simulink model "DCmotor_duo_PID_control_inter_position"  (R2023a)
settings: Solver=VariableStepAuto  StartTime=0.0  StopTime=inf  FixedStep=0.001  MaxStep=1e-3
values from neighbouring files (symbols this model uses):
  S = S_simple    [setupModelParameters.m]
undefined symbols (not defined in the file or in its folder): dval, ival, pval
libraries: slpidlib x1
settings Model: Creator=jamess  LastModifiedBy=leoyi
settings SolverCC: AlgebraicLoopSolver=TrustRegion
settings DataIOCC: ReturnWorkspaceOutputs=off
settings OptimizationCC: LifeSpan=inf
settings DebuggingCC: UnconnectedInputMsg=warning  UnconnectedOutputMsg=warning  UnconnectedLineMsg=warning  ArithmeticOperatorsInVariantConditions=warning
settings ModelReferenceCC: EnableRefExpFcnMdlSchedulingChecks=on
settings SFSimCC: SimUseLocalCustomCode=off  CustomCodeUndefinedFunction=UseInterfaceOnly
settings RTWCC: RTWUseLocalCustomCode=off
settings CodeAppCC: StateflowObjectComments=on

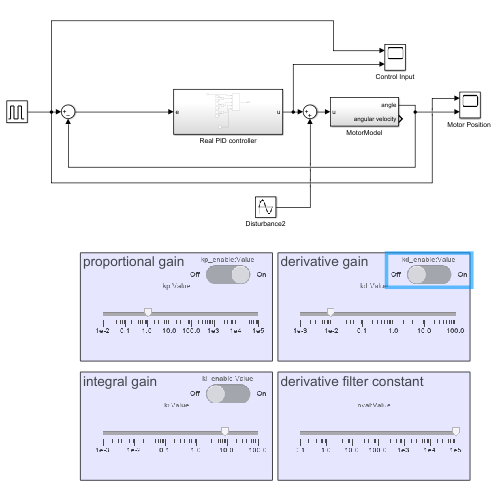
[thumbnail: Simulink's stored preview of the top-level diagram]
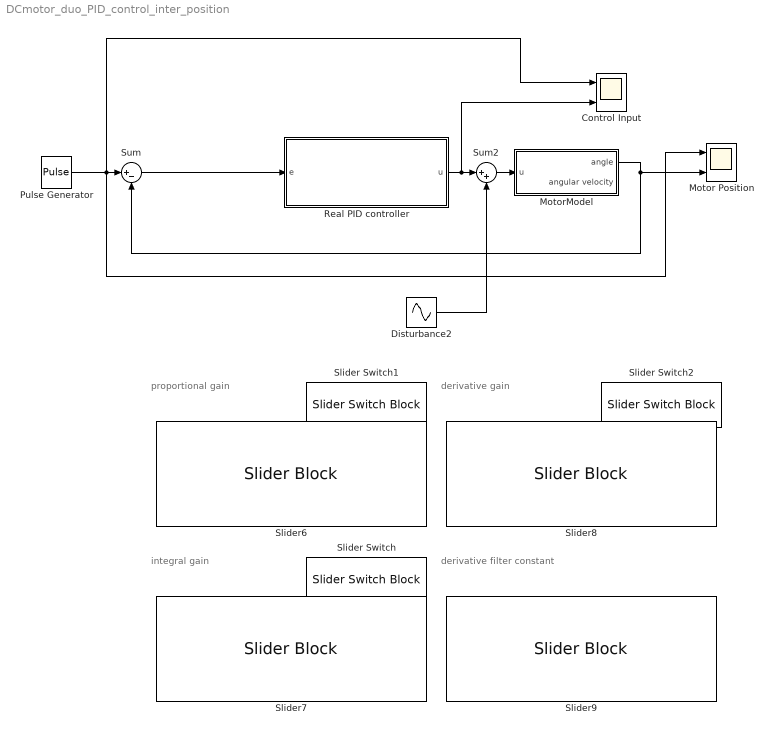
== system DCmotor_duo_PID_control_inter_position ==
  note: derivative gain
  note: proportional gain
  note: integral gain
  note: derivative filter constant
  Control Input : Scope  NumInputPorts=2
  Disturbance2 : Sin  Amplitude=0  Frequency=10*2*pi  SampleTime=0
  "Motor Position " : Scope  NumInputPorts=2
  MotorModel : Subsystem
  Pulse Generator : DiscretePulseGenerator  PulseType=Time based  Period=10  PulseWidth=50  PhaseDelay=0.1
  Real PID controller : Subsystem
  Slider Switch : SliderSwitchBlock
      settings: Values={{'Off', 'On'}, [0 1]}
  Slider Switch1 : SliderSwitchBlock
      settings: Values={{'Off', 'On'}, [0 1]}
  Slider Switch2 : SliderSwitchBlock
      settings: Values={{'Off', 'On'}, [0 1]}
  Slider6 : SliderBlock  ScaleMin=0.01  ScaleMax=100000  ScaleType=Log
  Slider7 : SliderBlock  ScaleMin=0.001  ScaleType=Log
  Slider8 : SliderBlock  ScaleMin=0.001  ScaleType=Log
  Slider9 : SliderBlock  ScaleMin=0.1  ScaleMax=1e5  ScaleType=Log
  Sum : Sum  Inputs=|+-
  Sum2 : Sum  Inputs=|++
  wires:
  MotorModel/1(angle) -> "Motor Position "/2, Sum/2
  Real PID controller/1(u) -> Control Input/2, Sum2/1
  Sum2/1 -> MotorModel/1(u)
  Pulse Generator/1 -> Control Input/1, "Motor Position "/1, Sum/1
  Disturbance2/1 -> Sum2/2
  Sum/1 -> Real PID controller/1(e)

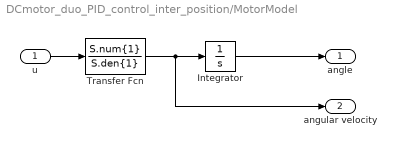
== system DCmotor_duo_PID_control_inter_position/MotorModel ==
  u : Inport
  Integrator : Integrator
  Transfer Fcn : TransferFcn  Numerator=S.num{1}  Denominator=S.den{1}
  angle : Outport
  angular velocity : Outport  Port=2
  wires:
  u/1 -> Transfer Fcn/1
  Transfer Fcn/1 -> angular velocity/1, Integrator/1
  Integrator/1 -> angle/1

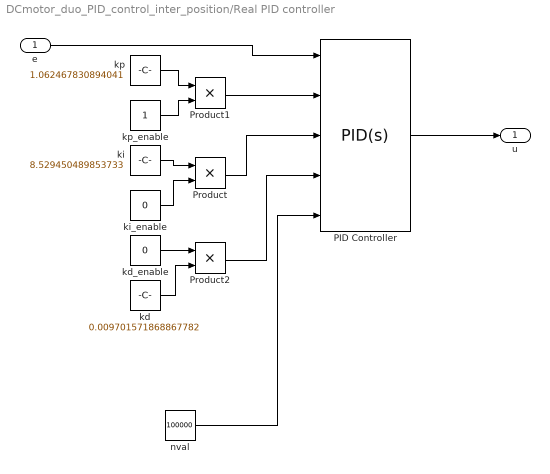
== system DCmotor_duo_PID_control_inter_position/Real PID controller ==
  e : Inport
  PID Controller : slpidlib/PID Controller  Controller=PID  Form=Parallel  TimeDomain=Continuous-time  UseExternalTs=off  SampleTime=-1  IntegratorMethod=Forward Euler  FilterMethod=Forward Euler  ControllerParametersSource=external  P=pval  I=ival  UseKiTs=off  D=dval  N=100  UseFilter=on  TunerSelectOption=Transfer Function Based (PID Tuner App)  InitialConditionSource=internal  InitialConditionForIntegrator=0  InitialConditionForFilter=0  DifferentiatorICPrevScaledInput=0  ExternalReset=none  TrackingMode=off  Kt=1  LimitOutput=off  SatLimitsSource=internal  UpperSaturationLimit=inf  LowerSaturationLimit=-inf  LinearizeAsGain=on  AntiWindupMode=none  Kb=1  LimitIntegrator=off  UpperIntegratorSaturationLimit=inf  LowerIntegratorSaturationLimit=-inf  POutMin=[]  POutMax=[]  IOutMin=[]  IOutMax=[]  DOutMin=[]  DOutMax=[]  NOutMin=[]  NOutMax=[]  SumOutMin=[]  SumOutMax=[]  SaturationOutMin=[]  SaturationOutMax=[]  PParamMin=[]  PParamMax=[]  IParamMin=[]  IParamMax=[]  DParamMin=[]  DParamMax=[]  NParamMin=[]  NParamMax=[]  KbParamMin=[]  KbParamMax=[]  KtParamMin=[]  KtParamMax=[]  KbOutMin=[]  KbOutMax=[]  KtOutMin=[]  KtOutMax=[]  IntegratorOutMin=[]  IntegratorOutMax=[]  FilterOutMin=[]  FilterOutMax=[]  SumI1OutMin=[]  SumI1OutMax=[]  SumI2OutMin=[]  SumI2OutMax=[]  SumI3OutMin=[]  SumI3OutMax=[]  SumI4OutMin=[]  SumI4OutMax=[]  SumDOutMin=[]  SumDOutMax=[]  DifferentiatorOutMin=[]  DifferentiatorOutMax=[]  FilterDiffOutCoefMin=[]  FilterDiffOutCoefMax=[]  ReciprocalOutMin=[]  ReciprocalOutMax=[]  SumDenOutMin=[]  SumDenOutMax=[]  SumNumOutMin=[]  SumNumOutMax=[]  DivideOutMin=[]  DivideOutMax=[]  UdiffTsProdOutMin=[]  UdiffTsProdOutMax=[]  NTsProdOutMin=[]  NTsProdOutMax=[]  UintegralTsProdOutMin=[]  UintegralTsProdOutMax=[]  UngainTsProdOutMin=[]  UngainTsProdOutMax=[]  ClampingZeroOutDataTypeStr=Inherit: Inherit via back propagation  ClampingZeroOutMin=[]  ClampingZeroOutMax=[]  FilterDenConstantOutDataTypeStr=Inherit: Inherit via back propagation  FilterDenConstantOutMin=[]  FilterDenConstantOutMax=[]  PCopyOutDataTypeStr=Inherit: Inherit via back propagation  PCopyOutMin=[]  PCopyOutMax=[]  NCopyOutDataTypeStr=Inherit: Inherit via back propagation  NCopyOutMin=[]  NCopyOutMax=[]  IntegratorContinuousStateAttributes=''  IntegratorStateMustResolveToSignalObject=off  IntegratorRTWStateStorageClass=Auto  FilterContinuousStateAttributes=''  FilterStateMustResolveToSignalObject=off  FilterRTWStateStorageClass=Auto  ParallelPVariant=ExternalParameters  IdealPVariant=Disabled  IVariant=ExternalParameters  DVariant=ExternalParameters  IntegratorVariant=Continuous  SatVariant=Disabled  AWVariant=Passthrough  PCopyVariant=Disabled  TRVariant=Disabled  FdbkBlocksVariant=Forward  IdealPFdbkVariant=Disabled  SatFdbkVariant=Disabled  DerivativeFilterVariant=ContFilter  NVariant=ExternalParameters  NCopyVariant=Disabled  FilterICVariant=InternalICsFilter  IntegratorICVariant=InternalICs  ExternalResetVariant=Disabled  TRSumVariant=Passthrough  SumFdbkVariant=Disabled  SumVariant=Sum_PID  TsampFilterVariant=InternalTs  TsampNgainVariant=Passthrough  TsampIntegralVariant=Disabled_SignalSpec  ExternalSaturationOutDataTypeStr=Inherit: Same as second input
  Product : Product
  Product1 : Product
  Product2 : Product
  kd : Constant  Value=0.009701571868867782
  kd_enable : Constant  Value=0
  ki : Constant  Value=8.529450489853733
  ki_enable : Constant  Value=0
  kp : Constant  Value=1.062467830894041
  kp_enable : Constant
  nval : Constant  Value=100000
  u : Outport
  wires:
  e/1 -> PID Controller/1
  nval/1 -> PID Controller/5
  PID Controller/1 -> u/1
  ki/1 -> Product/1
  Product/1 -> PID Controller/3
  ki_enable/1 -> Product/2
  kp_enable/1 -> Product1/2
  kp/1 -> Product1/1
  Product1/1 -> PID Controller/2
  kd_enable/1 -> Product2/1
  kd/1 -> Product2/2
  Product2/1 -> PID Controller/4
